simulink model "Traffic_light_control"  (R2020b)
settings: Solver=VariableStepAuto  StartTime=0.0  StopTime=10.0  RelTol=1e-3
settings Model: Creator=153  LastModifiedBy=153

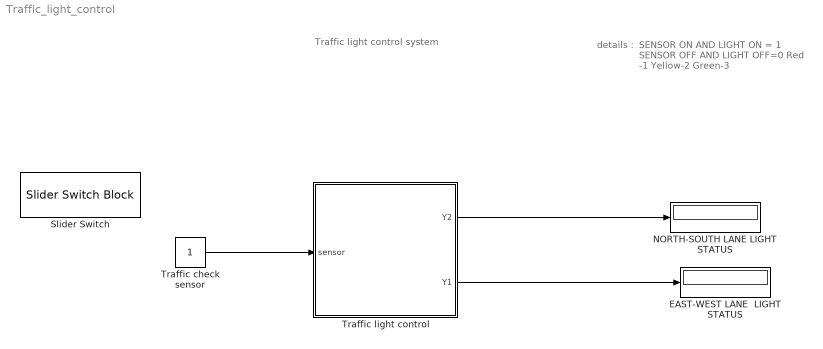
== system Traffic_light_control ==
  note: SENSOR ON AND LIGHT ON = 1
      | SENSOR OFF AND LIGHT OFF=0
      | Red -1
      | Yellow-2
      | Green-3
  note: details :
  note: Traffic light control system
  EAST-WEST LANE  LIGHT STATUS : Display
  NORTH-SOUTH LANE LIGHT STATUS : Display
  Slider Switch : SliderSwitchBlock
      settings: Values={{'Off', 'On'}, [0 1]}
  "Traffic check sensor " : Constant
  "Traffic light control " : Stateflow chart  TreatAsAtomicUnit=on
  wires:
  "Traffic light control "/1(Y2) -> NORTH-SOUTH LANE LIGHT STATUS/1
  "Traffic light control "/2(Y1) -> EAST-WEST LANE  LIGHT STATUS/1
  "Traffic check sensor "/1 -> "Traffic light control "/1(sensor)

== stateflow chart Traffic_light_control/Traffic light control  ==
  settings: stateMachineType=MOORE_MACHINE
  state stopfortraffic
    Y1=RED;
    Y2=GREEN;
  state stoptogo
    Y1=RED;
    Y2=YELLOW;
  state stop
    Y1=RED;
    Y2=GREEN;
  state gotostop
    Y1=YELLOW;
    Y2=RED;
  state go
    Y1=GREEN;
    Y2=RED;
  (default) -> stop
  stopfortraffic -> stoptogo : [sensor==1]
  stop -> stopfortraffic : after(20,tick)
  gotostop -> stop : after(3,tick)
  stoptogo -> go : after(3,tick)
  go -> gotostop : after(10,tick)
  data: RED constant double =1; YELLOW constant double =2; GREEN constant double =3; Y2 output; Y1 output; sensor input
